simulink model "MMC_Control_PLECS_IFB_simplify_ab0"  (R2016a)
settings: Solver=VariableStepAuto  SolverMode=SingleTasking  StartTime=0.0  StopTime=0.08  FixedStep=sim_Ts  RelTol=1e-3
undefined symbols (not defined in the file or in its folder): I25, plecs, V25
settings Model: Creator=jason  LastModifiedBy=Francis Chen
settings DebuggingCC: SFUnexpectedBacktrackingDiag=error  SFNoUnconditionalDefaultTransitionDiag=error
settings SFSimCC: SimUseLocalCustomCode=on
settings RTWCC: RTWUseLocalCustomCode=on
settings GRTTargetCC: TargetLangStandard=C99 (ISO)  GeneratePreprocessorConditionals=Use local settings
settings ConfigComp: CovMetricSettings=dwe  CovHtmlReporting=off  CovSaveCumulativeToWorkspaceVar=off  CovSaveSingleToWorkspaceVar=off  CovExternalEMLEnable=on

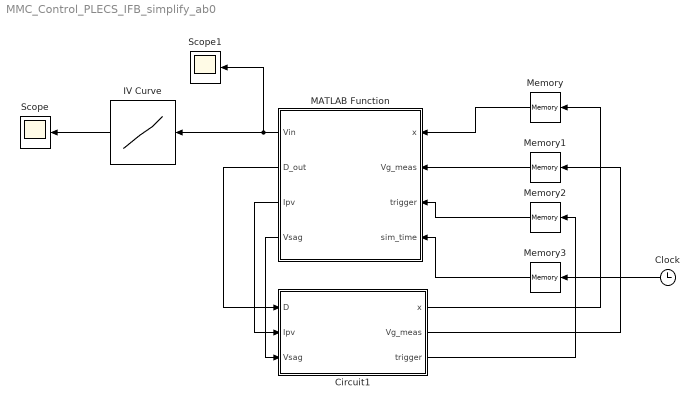
== system MMC_Control_PLECS_IFB_simplify_ab0 ==
  Circuit1 : Subsystem  LoadFcn=plecs('sl', 200);  InitFcn=plecs('sl', 214);  StartFcn=plecs('sl', 208);  StopFcn=plecs('sl', 209);  mask(PlecsCircuit){PLECSData=<binary blob, 39248 chars, not shown>}
      mask prompts: PLECSData "PLECS Data (Do not delete or modify!)"
      mask init:
      | % PLACE CUSTOM INITIALIZATIONS ABOVE
      | % DO NOT REMOVE
      | plecs('sl', 215);
      | % DO NOT REMOVE
      settings: CopyFcn=plecs('sl', 203);  DeleteFcn=plecs('sl', 205);  UndoDeleteFcn=plecs('sl', 206);  PreSaveFcn=plecs('sl', 211);  PostSaveFcn=plecs('sl', 201);  NameChangeFcn=plecs('sl', 210);  DestroyFcn=plecs('sl', 207);  PreCopyFcn=plecs('sl', 216);  OpenFcn=plecs('sl', 202);  ErrorFcn=plerrorfcn
      mask Help: web(['file:///' fullfile(plecsdoc, 'creatingacircuit.html')])
      mask Display: disp('PLECS\nCircuit')
  Clock : Clock
  IV Curve : Lookup_n-D  NumberOfTableDimensions=1  BreakpointsForDimension1=V25  Table=I25  ExtrapMethod=Clip  UseLastTableValue=on  InternalRulePriority=Speed  RndMeth=Simplest  InputSameDT=on
  MATLAB Function : MATLAB Function  TreatAsAtomicUnit=on
  Memory : Memory  X0=[50,50,50,4,4,4];  InheritSampleTime=on
  Memory1 : Memory  X0=[0,0,0];  InheritSampleTime=on
  Memory2 : Memory  InheritSampleTime=on
  Memory3 : Memory  InheritSampleTime=on
  Scope : Scope
  Scope1 : Scope
  wires:
  Circuit1/3(trigger) -> Memory2/1
  Circuit1/2(Vg_meas) -> Memory1/1
  Circuit1/1(x) -> Memory/1
  MATLAB Function/2(D_out) -> Circuit1/1(D)
  Memory/1 -> MATLAB Function/1(x)
  Memory1/1 -> MATLAB Function/2(Vg_meas)
  Memory2/1 -> MATLAB Function/3(trigger)
  MATLAB Function/1(Vin) -> Scope1/1, IV Curve/1
  IV Curve/1 -> Scope/1
  Clock/1 -> Memory3/1
  Memory3/1 -> MATLAB Function/4(sim_time)
  MATLAB Function/3(Ipv) -> Circuit1/2(Ipv)
  MATLAB Function/4(Vsag) -> Circuit1/3(Vsag)

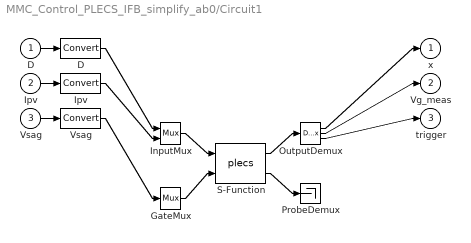
== system MMC_Control_PLECS_IFB_simplify_ab0/Circuit1 ==
  D : Inport  PortDimensions=6
  Ipv : Inport  Port=2  PortDimensions=3
  Vsag : Inport  Port=3  PortDimensions=1
  " D " : DataTypeConversion  SaturateOnIntegerOverflow=on  RndMeth=Zero
  " GateMux " : Mux  Inputs=[ 1 ]
  " InputMux " : Mux  Inputs=[ 6 3 ]
  " Ipv " : DataTypeConversion  SaturateOnIntegerOverflow=on  RndMeth=Zero
  " OutputDemux " : Demux  Outputs=[ 6 3 1 ]
  " ProbeDemux " : Terminator
  " S-Function " : S-Function  FunctionName=plecs  SFunctionDeploymentMode=off  EnableBusSupport=off
  " Vsag " : DataTypeConversion  SaturateOnIntegerOverflow=on  RndMeth=Zero
  x : Outport  PortDimensions=6
  Vg_meas : Outport  Port=2  PortDimensions=3
  trigger : Outport  Port=3  PortDimensions=1
  wires:
  " InputMux "/1 -> " S-Function "/1
  " GateMux "/1 -> " S-Function "/2
  " S-Function "/1 -> " OutputDemux "/1
  " S-Function "/2 -> " ProbeDemux "/1
  D/1 -> " D "/1
  " D "/1 -> " InputMux "/1
  Ipv/1 -> " Ipv "/1
  " Ipv "/1 -> " InputMux "/2
  Vsag/1 -> " Vsag "/1
  " Vsag "/1 -> " GateMux "/1
  " OutputDemux "/1 -> x/1
  " OutputDemux "/2 -> Vg_meas/1
  " OutputDemux "/3 -> trigger/1

== matlab function MMC_Control_PLECS_IFB_simplify_ab0/MATLAB Function ==
  data: Vin output; x input; D_out output; Vg_meas input; trigger input; sim_time input; nom parameter; Ipv output; Vsag output
function [Vin,D_out,Ipv,Vsag]  = MMC_control_AB0(x, Vg_meas, trigger, sim_time, nom)

persistent D_out_val err_int_val grid_angle_val Vg_peak fg phi
if isempty(D_out_val)
    grid_angle_val = 0;
    D_out_val = [0.5; 0.5; 0.5; 0.5; 0.5; 0.5];
    err_int_val = zeros(5,1);
    Vg_peak = nom.Vg_peak;
    fg = nom.fg ;
    phi = 0; 
end

if trigger    

Nstate = 6; 
Nout = 5; 
Kclark = 2/3*[1,-0.5,-0.5;0 sqrt(3)/2 -sqrt(3)/2;1/3,1/3,1/3]; %clark transform for ABC 

% assume open loop perfect phase measurement
grid_angle = mod( sim_time * fg * 2*pi+phi,2*pi ); 

if abs(sin(grid_angle))>0.1
Vg_peak = 0.9 * Vg_peak + 0.1* Vg_meas(1)/sin(grid_angle); %Complementery filter
end

tstep   = ceil(interp1(nom.phi,nom.id,grid_angle,'nearest','extrap'));
xnom    = nom.x(tstep,:)'; 

Ipv = interp1(nom.V25,nom.I25,x(1:3),'nearest','extrap'); 

Pin = sum(Ipv.*x(1:3)); 
Ig  = Pin*2/3/Vg_peak; 

phaseShift = 0;  
if sim_time>0.03 && sim_time < 0.08  
    phaseShift = pi/6; 
    Ig  = Pin*2/3/Vg_peak/cos(phaseShift);
end

xnom(4:6) = Kclark*[Ig*sin(grid_angle+phaseShift),Ig*sin(grid_angle-2*pi/3+phaseShift),Ig*sin(grid_angle+2*pi/3+phaseShift)]';

K       = nom.K(tstep,:,:);

xab       = [x(1:3);Kclark*x(4:6)]; %Clark Transformation to get the ab current
yab       = xab(1:5); 
yabd      = xnom(1:5); 

K  = reshape (K,Nstate,Nstate+Nout);
Ki = K       (:,1:Nout); 
Kp = K       (:,Nout+1:end);
tcy     = 1/nom.fsw;
D0      = nom.D (tstep,:)'; %Nominal Duty Cycle

state   =   xab - xnom; 
err     =   yabd - yab; 
err_int =   err*tcy  + err_int_val;

% Kp(1,2) = 0; Kp(1,3) = 0; 
% Kp(2,1) = 0; Kp(2,2) = 0; 
% Kp(3,2) = 0; Kp(3,3) = 0;
% Kp(4,1) = 0; Kp(4,3) = 0; 
% Kp(5,1) = 0; Kp(5,3) = 0; 
% Kp(6,1) = 0; Kp(6,2) = 0;
% 
% Ki(1,2) = 0; Ki(1,3) = 0; 
% Ki(2,1) = 0; Ki(2,2) = 0; 
% Ki(3,2) = 0; Ki(3,3) = 0;
% Ki(4,1) = 0; Ki(4,3) = 0; 
% Ki(5,1) = 0; Ki(5,3) = 0; 
% Ki(6,1) = 0; Ki(6,2) = 0;

dD      = - Kp*state - Ki*err_int;
D       =   D0+dD;  % pay close attention to the sign!
D       =   max(min(D,0.999),-0.999);
 
    D_out = D;
    D_out_val = D;
    err_int_val = err_int;
    grid_angle_val = grid_angle; 
else
    grid_angle = grid_angle_val; 
    D_out = D_out_val;
end
    Vin = x(1:3); 
    Ipv = interp1(nom.V25,nom.I25,x(1:3),'nearest','extrap'); 
    Vsag = 0; 
%     if sim_time>0.03
%         if sim_time > 0.06
% %             Vsag = 0;
% %             fg = 60; 
% %             phi = 0; 
%         else
%             Ipv(1) = Ipv(1)/2;
% %             Vsag = 1;
% %             phi = 1; 
% %             fg = 60; 
%         end
%     else
%         Vsag=0;
%     end
end %function
